simulink model "spring_damper_model"  (R2022b)
settings: Solver=VariableStepAuto  StartTime=0.0  StopTime=10.0  RelTol=1e-3
settings Model: Creator=Dharshan K  LastModifiedBy=Dharshan K

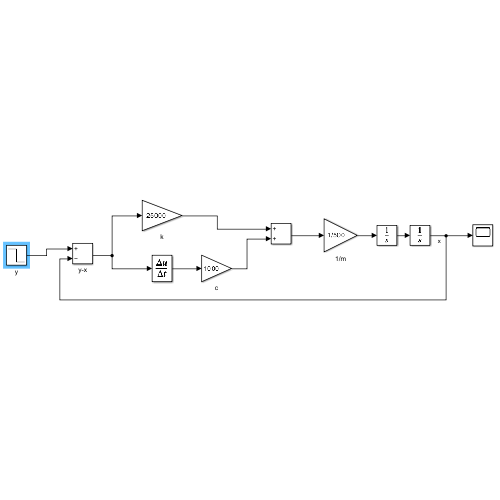
[thumbnail: Simulink's stored preview of the top-level diagram]
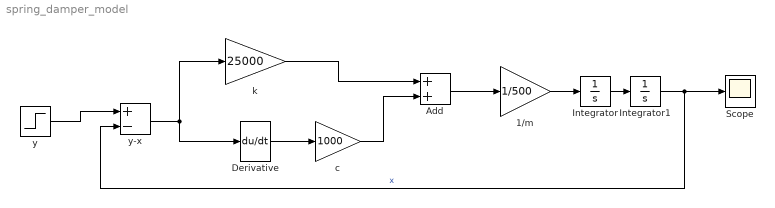
== system spring_damper_model ==
  1/m : Gain  Gain=1/500
  Add : Sum
  Derivative : Derivative
  Integrator : Integrator
  Integrator1 : Integrator
  Scope : Scope
  c : Gain  Gain=1000
  "k " : Gain  Gain=25000
  y : Step  Before=2  SampleTime=0
  y-x : Sum  Inputs=+-
  wires:
  y/1 -> y-x/1
  y-x/1 -> "k "/1, Derivative/1
  Derivative/1 -> c/1
  "k "/1 -> Add/1
  c/1 -> Add/2
  Add/1 -> 1/m/1
  1/m/1 -> Integrator/1
  Integrator/1 -> Integrator1/1
  Integrator1/1 -> y-x/2, Scope/1  "x"
